simulink model "gabor_simulation"  (Simulink 8.2)
settings: Solver=ode8  StartTime=0.0  StopTime=20  RelTol=1e-3
settings Model: Creator=petter  LastModifiedBy=petter
settings DataIOCC: SaveOutput=off  SaveTime=off
settings OptimizationCC: ExpressionDepthLimit=128
settings DebuggingCC: MultiTaskDSMMsg=warning  MultiTaskCondExecSysMsg=none  FcnCallInpInsideContextMsg=EnableAllAsError
settings RTWCC: IncludeERTFirstTime=on
settings GRTTargetCC: CombineOutputUpdateFcns=on  GRTInterface=off

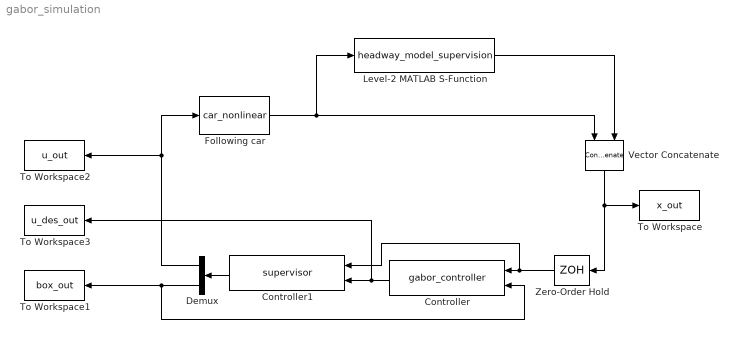
== system gabor_simulation ==
  Controller : M-S-Function  FunctionName=gabor_controller
  Controller1 : M-S-Function  FunctionName=supervisor  Parameters=1,3
  Demux : Demux  Outputs=2
  Following car : M-S-Function  FunctionName=car_nonlinear  Parameters=25
  Level-2 MATLAB S-Function : M-S-Function  FunctionName=headway_model_supervision  Parameters=90, 25
  To Workspace : ToWorkspace  VariableName=x_out  SampleTime=-1  SaveFormat=Structure With Time
  To Workspace1 : ToWorkspace  VariableName=box_out  SampleTime=-1  SaveFormat=Structure With Time
  To Workspace2 : ToWorkspace  VariableName=u_out  SampleTime=-1  SaveFormat=Structure With Time
  To Workspace3 : ToWorkspace  VariableName=u_des_out  SampleTime=-1  SaveFormat=Structure With Time
  Vector Concatenate : Concatenate
  Zero-Order Hold : ZeroOrderHold  SampleTime=0.1
  wires:
  Demux/1 -> To Workspace2/1, Following car/1
  Zero-Order Hold/1 -> Controller1/1, Controller/1
  Level-2 MATLAB S-Function/1 -> Vector Concatenate/2
  Vector Concatenate/1 -> Zero-Order Hold/1, To Workspace/1
  Following car/1 -> Level-2 MATLAB S-Function/1, Vector Concatenate/1
  Controller1/1 -> Demux/1
  Controller/1 -> To Workspace3/1, Controller1/2
  Demux/2 -> To Workspace1/1, Controller/2
